simulink subsystem "RoboRio_Controls_sub"  (R2023b)
settings: Solver=VariableStepAuto  StartTime=0.0  StopTime=10.0  RelTol=1e-3
libraries: Autonomous_lib x1, Disabled_lib x1, Teleop_lib x1, Test_lib x1
settings Model: Creator=USER  LastModifiedBy=FIRSTMentor

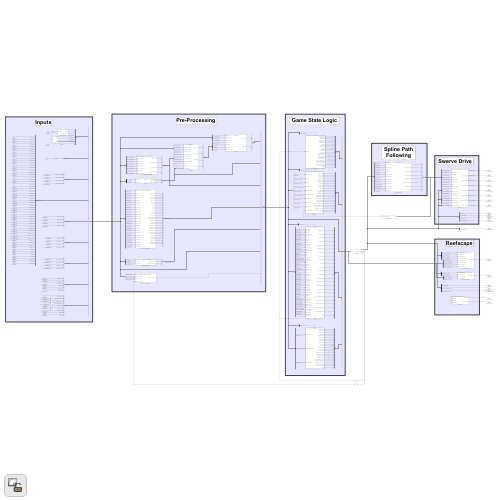
[thumbnail: Simulink's stored preview of the top-level diagram]
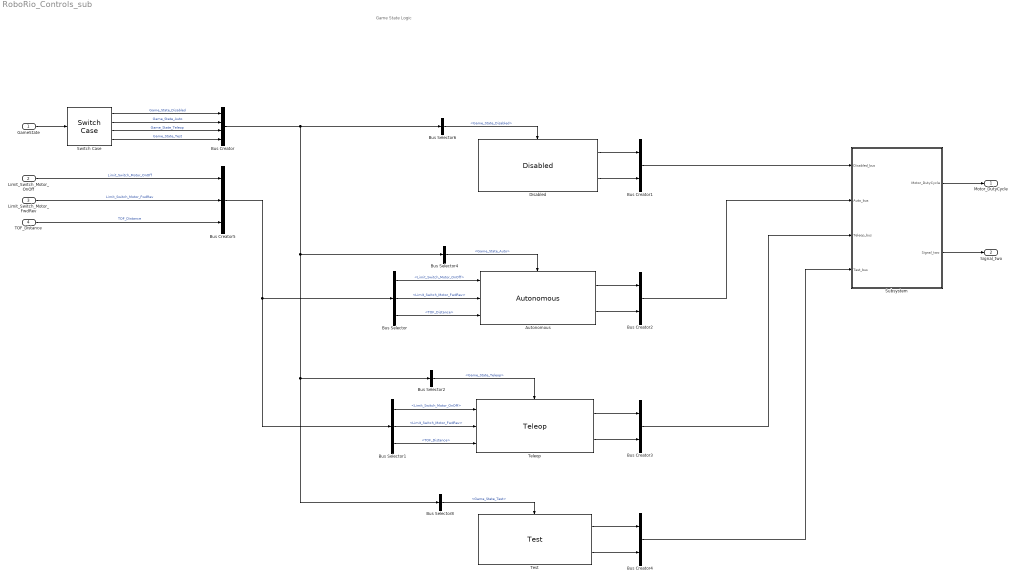
== system RoboRio_Controls_sub ==
  note: Game State Logic
  GameState : Inport
  Limit_Switch_Motor_OnOff : Inport  Port=2
  Limit_Switch_Motor_FwdRev : Inport  Port=3
  TOF_Distance : Inport  Port=4
  Autonomous : Autonomous_lib/Autonomous  SystemSampleTime=-1  VariantActivationTime=update diagram  AllowFlexibleInterface=on  Latency=0  AutoFrameSizeCalculation=off
  Bus Creator : BusCreator  Inputs=4
  Bus Creator{1..4} (4 alike) : BusCreator  Inputs=2
  Bus Creator5 : BusCreator  Inputs=3
  Bus Selector : BusSelector  OutputSignals=Limit_Switch_Motor_OnOff,Limit_Switch_Motor_FwdRev,TOF_Distance
  Bus Selector1 : BusSelector  OutputSignals=Limit_Switch_Motor_OnOff,Limit_Switch_Motor_FwdRev,TOF_Distance
  Bus Selector2 : BusSelector  OutputSignals=Game_State_Teleop
  Bus Selector4 : BusSelector  OutputSignals=Game_State_Auto
  Bus Selector6 : BusSelector  OutputSignals=Game_State_Disabled
  Bus Selector8 : BusSelector  OutputSignals=Game_State_Test
  Disabled : Disabled_lib/Disabled  SystemSampleTime=-1  VariantActivationTime=update diagram  AllowFlexibleInterface=on  Latency=0  AutoFrameSizeCalculation=off
  Subsystem : Subsystem
  Switch Case : SwitchCase  CaseConditions={0,1,2}
  Teleop : Teleop_lib/Teleop  SystemSampleTime=-1  VariantActivationTime=update diagram  AllowFlexibleInterface=on  Latency=0  AutoFrameSizeCalculation=off
  Test : Test_lib/Test  SystemSampleTime=-1  VariantActivationTime=update diagram  AllowFlexibleInterface=on  Latency=0  AutoFrameSizeCalculation=off
  Motor_DutyCycle : Outport
  Signal_two : Outport  Port=2
  wires:
  Bus Selector2/1 -> Teleop/Action  "<Game_State_Teleop>"
  Bus Selector4/1 -> Autonomous/Action  "<Game_State_Auto>"
  Bus Selector6/1 -> Disabled/Action  "<Game_State_Disabled>"
  Bus Selector8/1 -> Test/Action  "<Game_State_Test>"
  GameState/1 -> Switch Case/1
  Switch Case/1 -> Bus Creator/1  "Game_State_Disabled"
  Switch Case/2 -> Bus Creator/2  "Game_State_Auto"
  Switch Case/3 -> Bus Creator/3  "Game_State_Teleop"
  Switch Case/4 -> Bus Creator/4  "Game_State_Test"
  Bus Creator/1 -> Bus Selector6/1, Bus Selector4/1, Bus Selector2/1, Bus Selector8/1
  Disabled/1 -> Bus Creator1/1
  Disabled/2 -> Bus Creator1/2
  Autonomous/1 -> Bus Creator2/1
  Autonomous/2 -> Bus Creator2/2
  Teleop/1 -> Bus Creator3/1
  Teleop/2 -> Bus Creator3/2
  Test/1 -> Bus Creator4/1
  Test/2 -> Bus Creator4/2
  Limit_Switch_Motor_OnOff/1 -> Bus Creator5/1  "Limit_Switch_Motor_OnOff"
  Limit_Switch_Motor_FwdRev/1 -> Bus Creator5/2  "Limit_Switch_Motor_FwdRev"
  TOF_Distance/1 -> Bus Creator5/3  "TOF_Distance"
  Bus Selector/1 -> Autonomous/1  "<Limit_Switch_Motor_OnOff>"
  Bus Selector/2 -> Autonomous/2  "<Limit_Switch_Motor_FwdRev>"
  Bus Selector/3 -> Autonomous/3  "<TOF_Distance>"
  Bus Creator5/1 -> Bus Selector/1, Bus Selector1/1
  Bus Selector1/2 -> Teleop/2  "<Limit_Switch_Motor_FwdRev>"
  Bus Selector1/3 -> Teleop/3  "<TOF_Distance>"
  Bus Selector1/1 -> Teleop/1  "<Limit_Switch_Motor_OnOff>"
  Bus Creator1/1 -> Subsystem/1(Disabled_bus)
  Bus Creator2/1 -> Subsystem/2(Auto_bus)
  Bus Creator3/1 -> Subsystem/3(Teleop_bus)
  Bus Creator4/1 -> Subsystem/4(Test_bus)
  Subsystem/1(Motor_DutyCycle) -> Motor_DutyCycle/1
  Subsystem/2(Signal_two) -> Signal_two/1

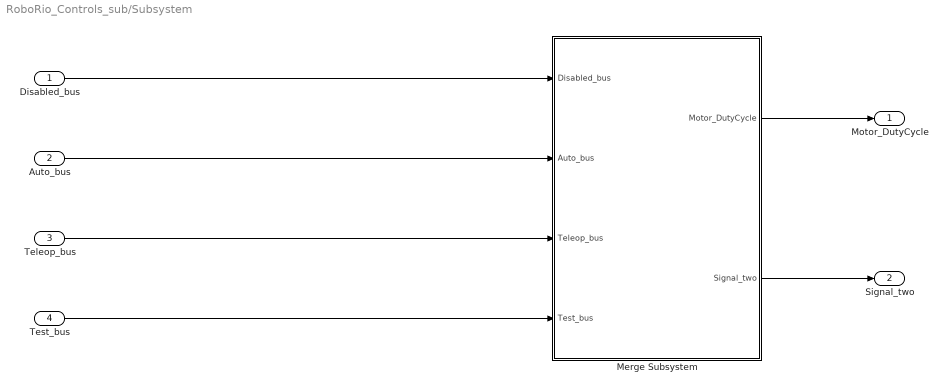
== system RoboRio_Controls_sub/Subsystem ==
  Disabled_bus : Inport
  Auto_bus : Inport  Port=2
  Teleop_bus : Inport  Port=3
  Test_bus : Inport  Port=4
  Merge Subsystem : Subsystem
  Motor_DutyCycle : Outport
  Signal_two : Outport  Port=2
  wires:
  Teleop_bus/1 -> Merge Subsystem/3(Teleop_bus)
  Auto_bus/1 -> Merge Subsystem/2(Auto_bus)
  Merge Subsystem/2(Signal_two) -> Signal_two/1
  Merge Subsystem/1(Motor_DutyCycle) -> Motor_DutyCycle/1
  Disabled_bus/1 -> Merge Subsystem/1(Disabled_bus)
  Test_bus/1 -> Merge Subsystem/4(Test_bus)

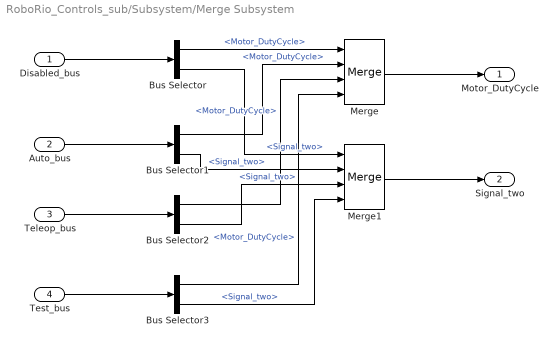
== system RoboRio_Controls_sub/Subsystem/Merge Subsystem ==
  Disabled_bus : Inport
  Auto_bus : Inport  Port=2
  Teleop_bus : Inport  Port=3
  Test_bus : Inport  Port=4
  Bus Selector{,1..3} (4 alike) : BusSelector  OutputSignals=Motor_DutyCycle,Signal_two
  Merge : Merge  Inputs=4
  Merge1 : Merge  Inputs=4
  Motor_DutyCycle : Outport
  Signal_two : Outport  Port=2
  wires:
  Bus Selector/1 -> Merge/1  "<Motor_DutyCycle>"
  Bus Selector3/2 -> Merge1/4  "<Signal_two>"
  Bus Selector2/2 -> Merge1/3  "<Signal_two>"
  Bus Selector1/2 -> Merge1/2  "<Signal_two>"
  Bus Selector/2 -> Merge1/1  "<Signal_two>"
  Merge1/1 -> Signal_two/1
  Merge/1 -> Motor_DutyCycle/1
  Bus Selector3/1 -> Merge/4  "<Motor_DutyCycle>"
  Bus Selector2/1 -> Merge/3  "<Motor_DutyCycle>"
  Bus Selector1/1 -> Merge/2  "<Motor_DutyCycle>"
  Test_bus/1 -> Bus Selector3/1
  Teleop_bus/1 -> Bus Selector2/1
  Auto_bus/1 -> Bus Selector1/1
  Disabled_bus/1 -> Bus Selector/1
